simulink model "test"  (R2019b)
settings: Solver=FixedStepAuto  StartTime=0.0  StopTime=1  RelTol=1e-3
undefined symbols (not defined in the file): F, Light, MIL
libraries: aerolibwind2 x1, sharedtransform x1
settings Model: Creator=Алексей  LastModifiedBy=Алексей
settings RTWCC: GenCodeOnly=on  PackageGeneratedCodeAndArtifacts=on

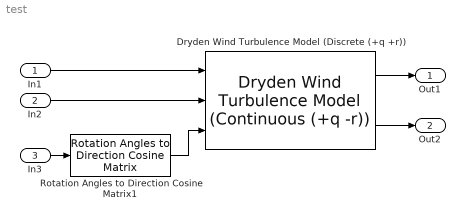
== system test ==
  In1 : Inport
  In2 : Inport  Port=2
  In3 : Inport  Port=3
  Dryden Wind Turbulence Model (Discrete (+q +r)) : aerolibwind2/Dryden Wind Turbulence Model  (Continuous (+q -r))  units=Metric (MKS)  spec=MIL-F-8785C  model=Discrete Dryden (+q +r)  W20=15  Wdeg=0  TurbProb=10^-2 - Light  L_high=533.4  Wingspan=10  ts=0.1  Seed=[23341 23342 23343 23344]  T_on=on
      settings: SourceProductName=Aerospace Blockset
  Rotation Angles to Direction Cosine Matrix1 : sharedtransform/Rotation Angles to Direction Cosine Matrix  rotationOrder=ZYX  aMode=aMode
      settings: SourceProductBaseCode=AE
  Out1 : Outport
  Out2 : Outport  Port=2
  wires:
  In3/1 -> Rotation Angles to Direction Cosine Matrix1/1
  Rotation Angles to Direction Cosine Matrix1/1 -> Dryden Wind Turbulence Model (Discrete (+q +r))/3
  In2/1 -> Dryden Wind Turbulence Model (Discrete (+q +r))/2
  Dryden Wind Turbulence Model (Discrete (+q +r))/1 -> Out1/1
  In1/1 -> Dryden Wind Turbulence Model (Discrete (+q +r))/1
  Dryden Wind Turbulence Model (Discrete (+q +r))/2 -> Out2/1
